simulink model "mloc_debug_mes"  (R2018b)
settings: configuration reference "Active" (kept outside this file)
undefined symbols (not defined in the file): tS
libraries: simulink x1
settings Model: DataDictionary=mloc_debug_mes.sldd  Creator=wischnewski  LastModifiedBy=ge34qer

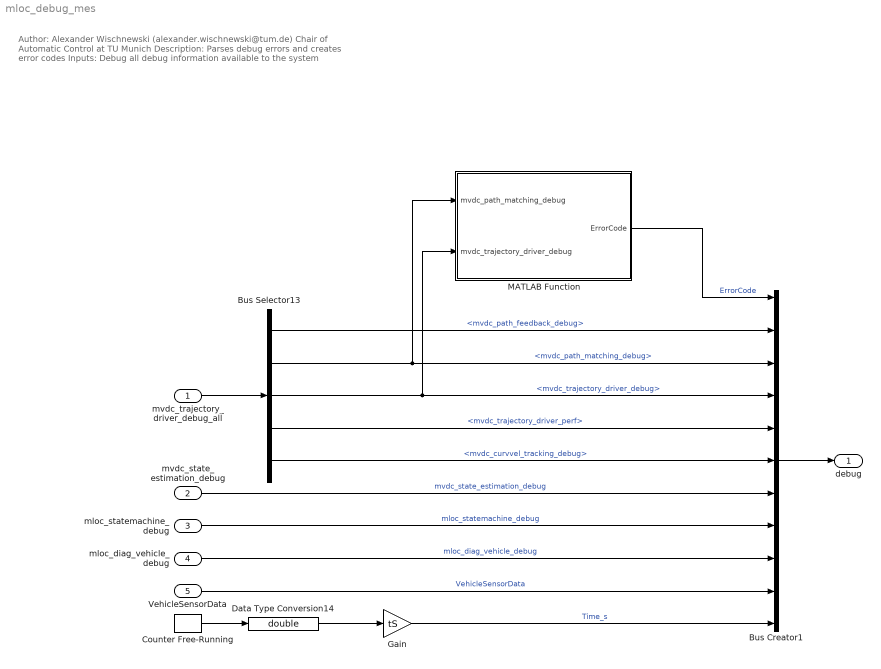
== system mloc_debug_mes ==
  note: Author: Alexander Wischnewski (alexander.wischnewski@tum.de)
      | Chair of Automatic Control at TU Munich
      |
      | Description: Parses debug errors and creates error codes
      |
      | Inputs:
      | Debug all debug information available to the system
  mvdc_trajectory_driver_debug_all : Inport  OutDataTypeStr=Bus: mvdc_trajectory_driver_debug_all
  mvdc_state_estimation_debug : Inport  Port=2  OutDataTypeStr=Bus: mvdc_state_estimation_debug
  mloc_statemachine_debug : Inport  Port=3  OutDataTypeStr=Bus: mloc_statemachine_debug
  mloc_diag_vehicle_debug : Inport  Port=4  OutDataTypeStr=Bus: mloc_diag_vehicle_debug
  VehicleSensorData : Inport  Port=5  OutDataTypeStr=Bus: VehicleSensorData
  Bus Creator1 : BusCreator  Inputs=11
  Bus Selector13 : BusSelector  OutputSignals=mvdc_path_feedback_debug,mvdc_path_matching_debug,mvdc_trajectory_driver_debug,mvdc_trajectory_driver_perf,mvdc_curvvel_tracking_debug
  Counter Free-Running : simulink/Sources/Counter Free-Running  NumBits=32  tsamp=tS
  Data Type Conversion14 : DataTypeConversion  OutDataTypeStr=double
  Gain : Gain  Gain=tS
  MATLAB Function : MATLAB Function  TreatAsAtomicUnit=on
  debug : Outport  OutDataTypeStr=Bus: mvdc_vehicle_dynamics_control_debug
  wires:
  VehicleSensorData/1 -> Bus Creator1/10  "VehicleSensorData"
  Bus Selector13/1 -> Bus Creator1/2  "<mvdc_path_feedback_debug>"
  Bus Selector13/4 -> Bus Creator1/5  "<mvdc_trajectory_driver_perf>"
  Counter Free-Running/1 -> Data Type Conversion14/1
  Bus Selector13/5 -> Bus Creator1/6  "<mvdc_curvvel_tracking_debug>"
  Bus Selector13/2 -> MATLAB Function/1(mvdc_path_matching_debug), Bus Creator1/3  "<mvdc_path_matching_debug>"
  mvdc_trajectory_driver_debug_all/1 -> Bus Selector13/1
  mloc_statemachine_debug/1 -> Bus Creator1/8  "mloc_statemachine_debug"
  Data Type Conversion14/1 -> Gain/1
  Bus Creator1/1 -> debug/1
  mloc_diag_vehicle_debug/1 -> Bus Creator1/9  "mloc_diag_vehicle_debug"
  Gain/1 -> Bus Creator1/11  "Time_s"
  Bus Selector13/3 -> MATLAB Function/2(mvdc_trajectory_driver_debug), Bus Creator1/4  "<mvdc_trajectory_driver_debug>"
  mvdc_state_estimation_debug/1 -> Bus Creator1/7  "mvdc_state_estimation_debug"
  MATLAB Function/1(ErrorCode) -> Bus Creator1/1  "ErrorCode"

== matlab function mloc_debug_mes/MATLAB Function ==
  data: mvdc_path_matching_debug input Bus: mvdc_path_matching_debug; ErrorCode output uint32; mvdc_trajectory_driver_debug input Bus: mvdc_trajectory_driver_debug
function ErrorCode = parseDebugSignals(mvdc_path_matching_debug, mvdc_trajectory_driver_debug)

ErrorCode = parseDebugSignals(mvdc_path_matching_debug, mvdc_trajectory_driver_debug);
